simulink model "leftLaneChangeRestructuredTest"  (R2019b)
settings: Solver=FixedStepAuto  StartTime=0.0  StopTime=10.0  FixedStep=Ts_bp  RelTol=1e-3
values from neighbouring files (symbols this model uses):
  P_init = .001    (= 0.001)    [initialization.m]
  rel_x = 0    [initialization.m]
  Ts_bp = 0.1    [initialization.m]    (also in laneChangeSinusoidalFcn.m = 0.01; laneChangeSinusoidalJacobianFcn.m = 0.01; leftLaneChangeParametricFcn.m; leftLaneChangeParametricWithAccFcn.m = 0.01)
  vx = X(2)    [cv_model_fun.m]    (also in initialization.m = 10)
  vy = X(4)    [cv_model_fun.m]    (also in initialization.m = 0)
  x = X(1)    [KinematicBicycleModel.m]    (also in SimplifiedKinematicBicycleModel.m; behavior_model.m = 0:0.01:20; cca_model_fun.m; ctra_model_fun.m)
  y = X(2)    [KinematicBicycleModel.m]    (also in SimplifiedKinematicBicycleModel.m; behavior_model.m = [distances velocities]; cca_model_fun.m; ctra_model_fun.m)
undefined symbols (not defined in the file or in its folder): sigbuilder_block
libraries: simulink x2
settings Model: Creator=jasprit  LastModifiedBy=jasprit

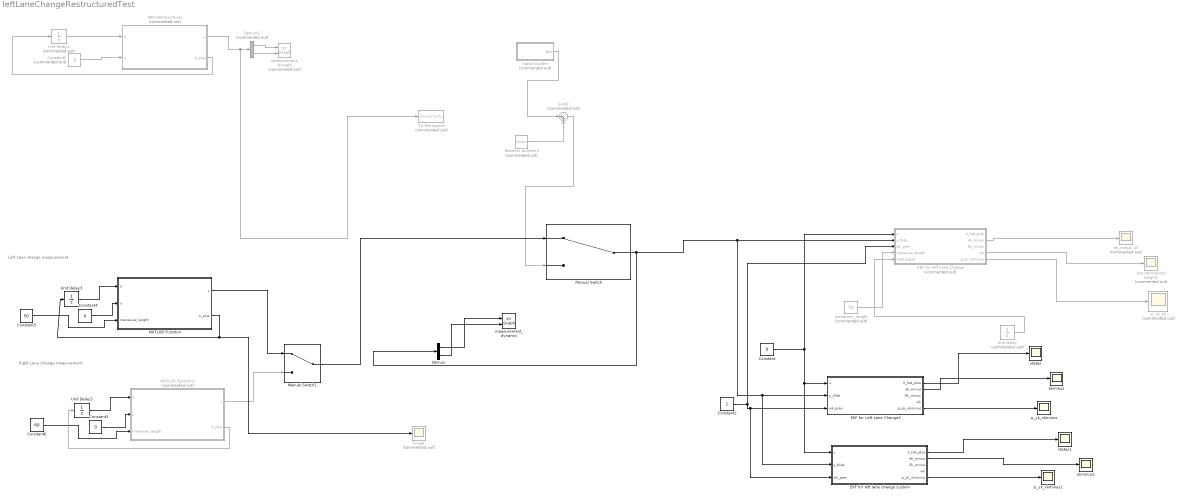
== system leftLaneChangeRestructuredTest ==
  note: Left Lane change measurement
  note: Right Lane Change measurement
  Constant : Constant  Value=0
  Constant1 : Constant  Value=0  SampleTime=-1
  Constant2 : Constant
  Constant3 : Constant  Value=50  SampleTime=-1
  Constant4 : Constant  Value=0  SampleTime=-1
  Constant5 : Constant  Commented=on  Value=0  SampleTime=-1
  Constant6 : Constant  Value=60
  Demux : Demux  Outputs=2
  Demux2 : Demux  Commented=on  Outputs=2
  EKF for Left Lane Change2 : Subsystem
  EKF for left Lane Change : Subsystem  Commented=on  TreatAsAtomicUnit=on
  EKF for left lane change custom : Subsystem
  MATLAB Function : MATLAB Function  TreatAsAtomicUnit=on
  MATLAB Function1 : MATLAB Function  Commented=on  TreatAsAtomicUnit=on
  MATLAB Function2 : MATLAB Function  Commented=on  TreatAsAtomicUnit=on
  Manual Switch : ManualSwitch
  Manual Switch1 : ManualSwitch
  Random Number2 : RandomNumber  Commented=on  Variance=0.0025  SampleTime=0.01
  Scope : Scope  Commented=on
  Signal Builder : Subsystem  Tag=STV Subsys  Commented=on  LoadFcn=sigbuilder_block('load');  StartFcn=sigbuilder_block('start');  StopFcn=sigbuilder_block('stop');  ClipboardFcn=sigbuilder_block('clipboard');  mask(Sigbuilder block){tuvar=[0:10]}
      mask help: Simulink:masks:SigbuilderBlock_MD
      mask init:
      | if ~strcmp(get_param(bdroot(gcbh),'SimulationStatus'),'stopped') tuvar = sigbuilder_block('maskInit'); end
      settings: CopyFcn=sigbuilder_block('copy');  DeleteFcn=sigbuilder_block('delete');  ModelCloseFcn=sigbuilder_block('modelClose');  PreSaveFcn=sigbuilder_block('preSave');  PauseFcn=sigbuilder_block('pause');  ContinueFcn=sigbuilder_block('continue');  NameChangeFcn=sigbuilder_block('namechange');  OpenFcn=sigbuilder_block('open',[418.5 99 558 422.25 ]);  CloseFcn=sigbuilder_block('close');
      mask Display: plot(0, 0, 100, 100,[2, 2, 32, 32, 2], [68, 8, 8, 68, 68],[32, 2], [38, 38], [32, 19, 2],[53, 60, 44], [32, 17, 17, 2],[16, 16, 31, 31]);txt = getActiveGroup(gcbh);text(2, 100, txt,'verticalAlignment', 'top');
  Sum2 : Sum  Commented=on  Inputs=|++
  To Workspace : ToWorkspace  Commented=on  VariableName=ground_truth_2  SaveFormat=Timeseries  SampleTime=-1
  Unit Delay : UnitDelay  Commented=on  SampleTime=-1  HasFrameUpgradeWarning=on
  Unit Delay3 : UnitDelay  InitialCondition=[x vx y vy]  SampleTime=Ts_bp  HasFrameUpgradeWarning=on
  Unit Delay4 : UnitDelay  Commented=on  InitialCondition=[x vx y vy]  SampleTime=-1  HasFrameUpgradeWarning=on
  Unit Delay5 : UnitDelay  InitialCondition=[x vx y vy]  SampleTime=Ts_bp  HasFrameUpgradeWarning=on
  ek_minus_All : Scope  Commented=on
  ekminus : Scope
  ekminus1 : Scope
  maneuver_length : Constant  Commented=on  Value=50
  measurement_dynamic : simulink/Sinks/XY Graph  xmin=-1  xmax=100  ymin=-5  ymax=5  st=-1
  measurement_straight : simulink/Sinks/XY Graph  Commented=on  xmin=-1  xmax=200  ymin=-5  ymax=5  st=-1
  p_yk_xk : Scope  Commented=on
  p_yk_xkminus : Scope
  p_yk_xkminus1 : Scope
  pre-normalized weights : Scope  Commented=on
  states : Scope
  states1 : Scope
  wires:
  Unit Delay3/1 -> MATLAB Function/1(X)
  MATLAB Function2/1(y) -> Manual Switch1/2
  Demux2/1 -> measurement_straight/1
  Constant/1 -> EKF for left lane change custom/1(u), EKF for Left Lane Change2/1(u), EKF for left Lane Change/1(u)
  Unit Delay5/1 -> MATLAB Function2/1(X)
  MATLAB Function1/1(y) -> To Workspace/1, Demux2/1
  Constant1/1 -> MATLAB Function2/2(u)
  Unit Delay/1 -> EKF for left Lane Change/5(reset signal)
  Constant2/1 -> EKF for left Lane Change/3(wk_prev), EKF for left lane change custom/3(wk_prev), EKF for Left Lane Change2/3(wk_prev)
  Constant6/1 -> MATLAB Function2/3(maneuver_length)
  MATLAB Function/1(y) -> Manual Switch1/1
  Manual Switch/1 -> EKF for left lane change custom/2(y_tilde), EKF for Left Lane Change2/2(y_tilde), EKF for left Lane Change/2(y_tilde), Demux/1
  Constant4/1 -> MATLAB Function/2(u)
  Unit Delay4/1 -> MATLAB Function1/1(X)
  Demux/1 -> measurement_dynamic/1
  Constant3/1 -> MATLAB Function/3(maneuver_length)
  MATLAB Function1/2(X_plus) -> Unit Delay4/1
  MATLAB Function/2(X_plus) -> Scope/1, Unit Delay3/1
  EKF for left Lane Change/5(p_yk_xkminus) -> p_yk_xk/1
  Sum2/1 -> Manual Switch/2
  Signal Builder/1(Bus) -> Sum2/1
  Random Number2/1 -> Sum2/2
  maneuver_length/1 -> EKF for left Lane Change/4(maneuver_length)
  EKF for left Lane Change/2(ek_minus) -> ek_minus_All/1
  Constant5/1 -> MATLAB Function1/2(u)
  MATLAB Function2/2(X_plus) -> Unit Delay5/1
  Demux2/2 -> measurement_straight/2
  Demux/2 -> measurement_dynamic/2
  EKF for left Lane Change/4(wk) -> pre-normalized weights/1
  Manual Switch1/1 -> Manual Switch/1
  EKF for Left Lane Change2/1(X_hat_plus) -> states/1
  EKF for Left Lane Change2/2(ek_minus) -> ekminus/1
  EKF for Left Lane Change2/5(p_yk_xkminus) -> p_yk_xkminus/1
  EKF for left lane change custom/2(ek_minus) -> ekminus1/1
  EKF for left lane change custom/1(X_hat_plus) -> states1/1
  EKF for left lane change custom/5(p_yk_xkminus) -> p_yk_xkminus1/1

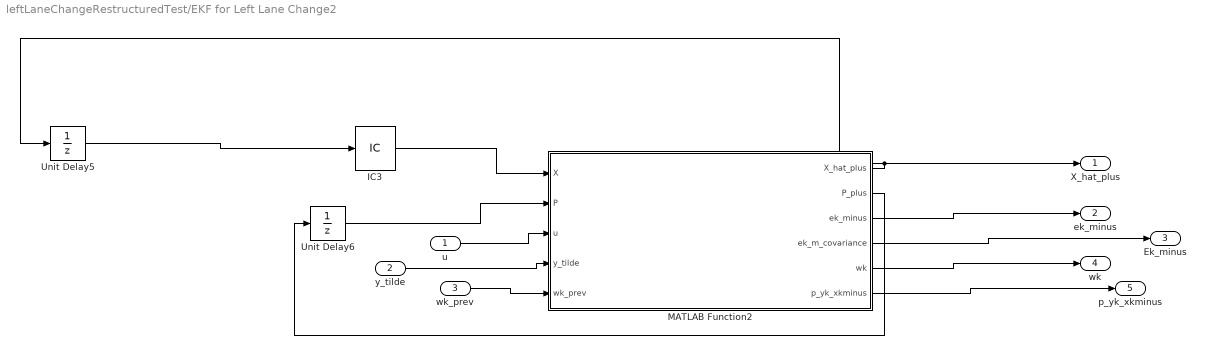
== system leftLaneChangeRestructuredTest/EKF for Left Lane Change2 ==
  u : Inport
  y_tilde : Inport  Port=2
  wk_prev : Inport  Port=3
  IC3 : InitialCondition  Value=[x vx y vy]
  MATLAB Function2 : MATLAB Function  TreatAsAtomicUnit=on
  Unit Delay5 : UnitDelay  SampleTime=-1  HasFrameUpgradeWarning=on
  Unit Delay6 : UnitDelay  InitialCondition=P_init  SampleTime=-1  HasFrameUpgradeWarning=on
  X_hat_plus : Outport  VectorParamsAs1DForOutWhenUnconnected=off
  ek_minus : Outport  Port=2  VectorParamsAs1DForOutWhenUnconnected=off
  Ek_minus : Outport  Port=3  VectorParamsAs1DForOutWhenUnconnected=off
  wk : Outport  Port=4  VectorParamsAs1DForOutWhenUnconnected=off
  p_yk_xkminus : Outport  Port=5  VectorParamsAs1DForOutWhenUnconnected=off
  wires:
  MATLAB Function2/2(P_plus) -> Unit Delay6/1
  u/1 -> MATLAB Function2/3(u)
  Unit Delay5/1 -> IC3/1
  y_tilde/1 -> MATLAB Function2/4(y_tilde)
  MATLAB Function2/1(X_hat_plus) -> Unit Delay5/1, X_hat_plus/1
  IC3/1 -> MATLAB Function2/1(X)
  Unit Delay6/1 -> MATLAB Function2/2(P)
  MATLAB Function2/3(ek_minus) -> ek_minus/1
  MATLAB Function2/4(ek_m_covariance) -> Ek_minus/1
  MATLAB Function2/5(wk) -> wk/1
  MATLAB Function2/6(p_yk_xkminus) -> p_yk_xkminus/1
  wk_prev/1 -> MATLAB Function2/5(wk_prev)

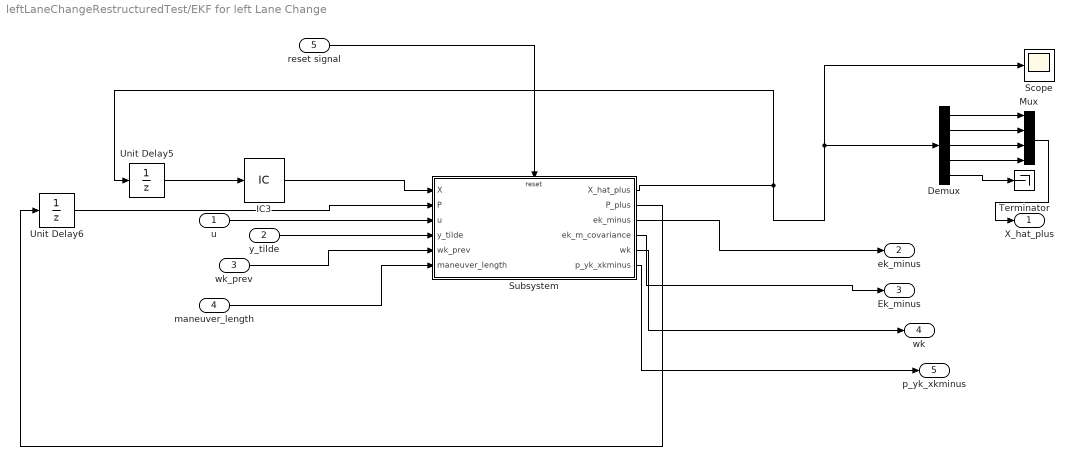
== system leftLaneChangeRestructuredTest/EKF for left Lane Change ==
  u : Inport
  y_tilde : Inport  Port=2
  wk_prev : Inport  Port=3
  maneuver_length : Inport  Port=4
  reset signal : Inport  Port=5
  Demux : Demux  Outputs=5
  IC3 : InitialCondition  Value=[x vx y vy rel_x]
  Mux : Mux
  Scope : Scope
  Subsystem : Subsystem
  Terminator : Terminator
  Unit Delay5 : UnitDelay  InitialCondition=[x vx y vy rel_x]  SampleTime=-1  HasFrameUpgradeWarning=on
  Unit Delay6 : UnitDelay  InitialCondition=diag([P_init, P_init, P_init, P_init, P_init])  SampleTime=-1  HasFrameUpgradeWarning=on
  X_hat_plus : Outport  VectorParamsAs1DForOutWhenUnconnected=off
  ek_minus : Outport  Port=2  VectorParamsAs1DForOutWhenUnconnected=off
  Ek_minus : Outport  Port=3  VectorParamsAs1DForOutWhenUnconnected=off
  wk : Outport  Port=4  VectorParamsAs1DForOutWhenUnconnected=off
  p_yk_xkminus : Outport  Port=5  VectorParamsAs1DForOutWhenUnconnected=off
  wires:
  Mux/1 -> X_hat_plus/1
  Demux/4 -> Mux/4
  Demux/5 -> Terminator/1
  Demux/3 -> Mux/3
  Demux/2 -> Mux/2
  Unit Delay5/1 -> IC3/1
  Demux/1 -> Mux/1
  Subsystem/1(X_hat_plus) -> Demux/1, Scope/1, Unit Delay5/1
  IC3/1 -> Subsystem/1(X)
  u/1 -> Subsystem/3(u)
  y_tilde/1 -> Subsystem/4(y_tilde)
  wk_prev/1 -> Subsystem/5(wk_prev)
  maneuver_length/1 -> Subsystem/6(maneuver_length)
  Subsystem/3(ek_minus) -> ek_minus/1
  Subsystem/4(ek_m_covariance) -> Ek_minus/1
  Subsystem/5(wk) -> wk/1
  Subsystem/6(p_yk_xkminus) -> p_yk_xkminus/1
  Unit Delay6/1 -> Subsystem/2(P)
  Subsystem/2(P_plus) -> Unit Delay6/1
  reset signal/1 -> Subsystem/Reset

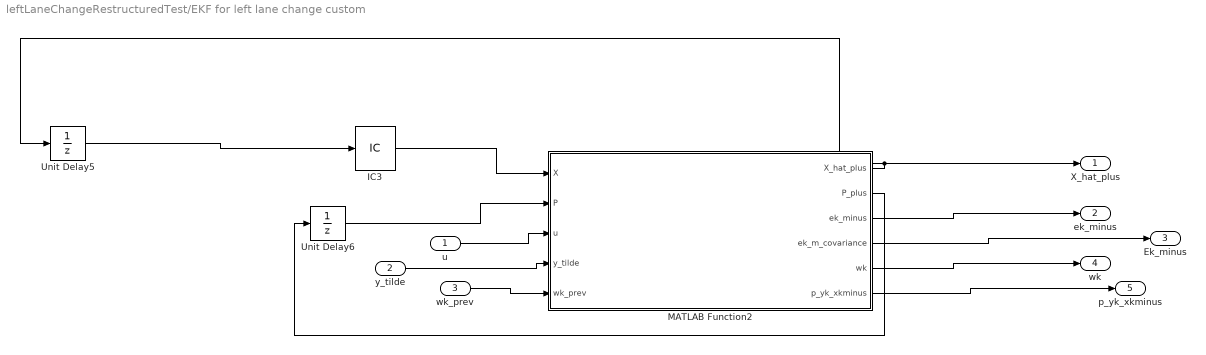
== system leftLaneChangeRestructuredTest/EKF for left lane change custom ==
  u : Inport
  y_tilde : Inport  Port=2
  wk_prev : Inport  Port=3
  IC3 : InitialCondition  Value=[x vx y vy]
  MATLAB Function2 : MATLAB Function  TreatAsAtomicUnit=on
  Unit Delay5 : UnitDelay  SampleTime=-1  HasFrameUpgradeWarning=on
  Unit Delay6 : UnitDelay  InitialCondition=P_init  SampleTime=-1  HasFrameUpgradeWarning=on
  X_hat_plus : Outport  VectorParamsAs1DForOutWhenUnconnected=off
  ek_minus : Outport  Port=2  VectorParamsAs1DForOutWhenUnconnected=off
  Ek_minus : Outport  Port=3  VectorParamsAs1DForOutWhenUnconnected=off
  wk : Outport  Port=4  VectorParamsAs1DForOutWhenUnconnected=off
  p_yk_xkminus : Outport  Port=5  VectorParamsAs1DForOutWhenUnconnected=off
  wires:
  MATLAB Function2/2(P_plus) -> Unit Delay6/1
  u/1 -> MATLAB Function2/3(u)
  Unit Delay5/1 -> IC3/1
  y_tilde/1 -> MATLAB Function2/4(y_tilde)
  MATLAB Function2/1(X_hat_plus) -> Unit Delay5/1, X_hat_plus/1
  IC3/1 -> MATLAB Function2/1(X)
  Unit Delay6/1 -> MATLAB Function2/2(P)
  MATLAB Function2/3(ek_minus) -> ek_minus/1
  MATLAB Function2/4(ek_m_covariance) -> Ek_minus/1
  MATLAB Function2/5(wk) -> wk/1
  MATLAB Function2/6(p_yk_xkminus) -> p_yk_xkminus/1
  wk_prev/1 -> MATLAB Function2/5(wk_prev)

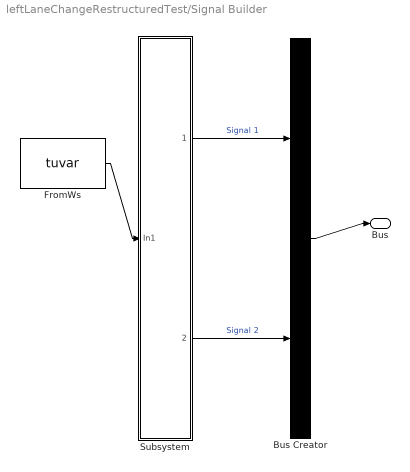
== system leftLaneChangeRestructuredTest/Signal Builder ==
  Bus Creator : BusCreator  Tag=Bus Creator  Inputs=2
  FromWs : FromWorkspace  Tag=STV FromWs  VariableName=tuvar  SampleTime=0
      SigBuilderData=|
      | common.afterFinalStr = 'Extrapolate'
      | common.sampleTime = 0
      | dataSet.timeRange = [0 20]
      | dataSet.name = 'Group 1'
      | sbobj.Groups.Name = 'Group 1'
      | sbobj.Groups.Signals(1).Name = 'Signal 1'
      | sbobj.Groups.Signals(1).XData = [0 0.01 0.02 0.03 0.04 0.05 0.06 0.07 0.08 0.09 0.1 0.11 ... (2001 elements, 1x2001)]
      | sbobj.Groups.Signals(1).YData = [0 0.1 0.2 0.3 0.4 0.5 0.6 0.7 0.8 0.9 1 1.1 ... (2001 elements, 1x2001)]
      | sbobj.Groups.Signals(2).Name = 'Signal 2'
      | sbobj.Groups.Signals(2).XData = [0 0.01 0.02 0.03 0.04 0.05 0.06 0.07 0.08 0.09 0.1 0.11 ... (2001 elements, 1x2001)]
      | sbobj.Groups.Signals(2).YData = [0 0 0 0 0 0 0 0 0 0 0 0 ... (2001 elements, 1x2001)]
      | sbobj.Groups.TimeRange = [0 20]
  Subsystem : Subsystem
  Bus : Outport  VectorParamsAs1DForOutWhenUnconnected=off
  wires:
  FromWs/1 -> Subsystem/1(In1)
  Bus Creator/1 -> Bus/1
  Subsystem/1(Signal 1) -> Bus Creator/1  "Signal 1"
  Subsystem/2(Signal 2) -> Bus Creator/2  "Signal 2"

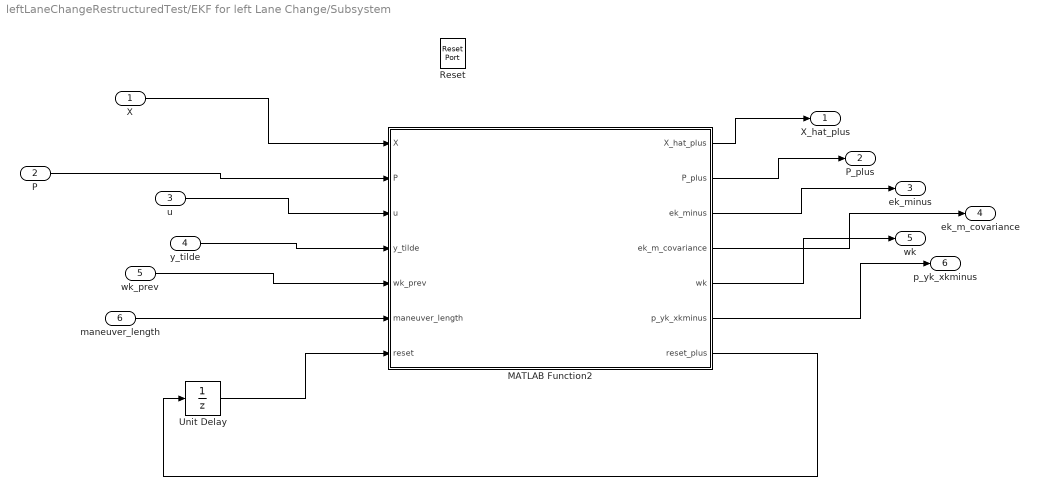
== system leftLaneChangeRestructuredTest/EKF for left Lane Change/Subsystem ==
  X : Inport
  P : Inport  Port=2
  u : Inport  Port=3
  y_tilde : Inport  Port=4
  wk_prev : Inport  Port=5
  maneuver_length : Inport  Port=6
  Reset : ResetPort  DisableCoverage=on
  MATLAB Function2 : MATLAB Function  TreatAsAtomicUnit=on
  Unit Delay : UnitDelay  InitialCondition=1  SampleTime=-1  HasFrameUpgradeWarning=on
  X_hat_plus : Outport  VectorParamsAs1DForOutWhenUnconnected=off
  P_plus : Outport  Port=2  VectorParamsAs1DForOutWhenUnconnected=off
  ek_minus : Outport  Port=3  VectorParamsAs1DForOutWhenUnconnected=off
  ek_m_covariance : Outport  Port=4  VectorParamsAs1DForOutWhenUnconnected=off
  wk : Outport  Port=5  VectorParamsAs1DForOutWhenUnconnected=off
  p_yk_xkminus : Outport  Port=6  VectorParamsAs1DForOutWhenUnconnected=off
  wires:
  MATLAB Function2/5(wk) -> wk/1
  MATLAB Function2/1(X_hat_plus) -> X_hat_plus/1
  X/1 -> MATLAB Function2/1(X)
  P/1 -> MATLAB Function2/2(P)
  u/1 -> MATLAB Function2/3(u)
  wk_prev/1 -> MATLAB Function2/5(wk_prev)
  MATLAB Function2/3(ek_minus) -> ek_minus/1
  y_tilde/1 -> MATLAB Function2/4(y_tilde)
  maneuver_length/1 -> MATLAB Function2/6(maneuver_length)
  MATLAB Function2/2(P_plus) -> P_plus/1
  MATLAB Function2/6(p_yk_xkminus) -> p_yk_xkminus/1
  MATLAB Function2/4(ek_m_covariance) -> ek_m_covariance/1
  Unit Delay/1 -> MATLAB Function2/7(reset)
  MATLAB Function2/7(reset_plus) -> Unit Delay/1

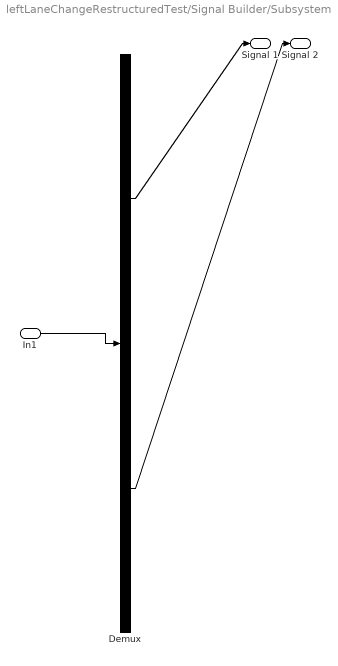
== system leftLaneChangeRestructuredTest/Signal Builder/Subsystem ==
  In1 : Inport
  Demux : Demux  Tag=STV Demux  Outputs=2
  Signal 1 : Outport  Tag=STV Outport  VectorParamsAs1DForOutWhenUnconnected=off
  Signal 2 : Outport  Tag=STV Outport  Port=2  VectorParamsAs1DForOutWhenUnconnected=off
  wires:
  In1/1 -> Demux/1
  Demux/1 -> Signal 1/1
  Demux/2 -> Signal 2/1

== matlab function leftLaneChangeRestructuredTest/EKF for Left Lane Change2/MATLAB Function2 ==
  data: X input; P input; u input; X_hat_plus output; y_tilde input; P_plus output; ek_minus output; ek_m_covariance output; wk output; p_yk_xkminus output; wk_prev input
function [X_hat_plus, P_plus, ek_minus, ek_m_covariance, wk, p_yk_xkminus] = EKFLeftLaneChangeCustom(X, P, u, y_tilde, wk_prev)

    maneuver_length = 50;  %meters
    lane_center_to_center_distance = 3.5;   %meters
    
    %%
    %TODO: See how can this be moved out of the function later
    %sampling time
    Ts = 0.1;

    % measurement noise covariance
%     R = [0.2 0; 0 0.2];
    R = [0.0025 0; 0 0.0025];
    
    % process noise covariance
%     Q = diag([0.5 5.0 0.5 5.0]);
    Q = diag([0.001 0.001 0.001 0.001]);

    % states - X = [x vx y vy] -     
    Ck = [1 0 0 0; 0 0 1 0];

    F = leftLaneChangeParametricJacobianFcn(X, u, maneuver_length, lane_center_to_center_distance);
    %%
    % Now estimate states using kalman filter
    
    %predict
    xhat_minus = leftLaneChangeParametricFcn(X, u, maneuver_length, lane_center_to_center_distance);
    P_minus = (F * P * F') + Ts*Q;
    yhat_minus = Ck * xhat_minus;

    %correct
    ek_minus = y_tilde - yhat_minus;    %residual
    ek_m_covariance = Ck * P_minus *Ck' + R;    %residual covariance
    K = P_minus * Ck' * inv(ek_m_covariance);
    X_hat_plus = xhat_minus + K * ek_minus;
    P_plus = (eye(4) - K * Ck) * P_minus;
    
    %calculate MMAE weights
    p_yk_xkminus = 1/sqrt(det(2*pi*ek_m_covariance))*exp(-1/2 * ek_minus'* inv(ek_m_covariance) * ek_minus);
    wk = wk_prev * p_yk_xkminus;

    
end

== matlab function leftLaneChangeRestructuredTest/EKF for left lane change custom/MATLAB Function2 ==
  data: X input; P input; u input; X_hat_plus output; y_tilde input; P_plus output; ek_minus output; ek_m_covariance output; wk output; p_yk_xkminus output; wk_prev input
function [X_hat_plus, P_plus, ek_minus, ek_m_covariance, wk, p_yk_xkminus] = EKFLeftLaneChangeCustom(X, P, u, y_tilde, wk_prev)

%%    
    persistent leftLCfilter;
    if isempty(leftLCfilter)
        maneuver_length = 50;  %meters
        lane_center_to_center_distance = 3.5;   %meters
        
        %TODO: See how can this be moved out of the function later
        %sampling time
        Ts = 0.1;
        
        mm = LeftLaneChangeSinusoidalMotionModel(Ts,maneuver_length, lane_center_to_center_distance);
        
        leftLCfilter = XKalmanFilter(Ts,mm);
        
        % measurement noise covariance
        %     R = [0.2 0; 0 0.2];
        R = [0.0025 0; 0 0.0025];
        
        % process noise covariance
        %     Q = diag([0.5 5.0 0.5 5.0]);
        Q = diag([0.001 0.001 0.001 0.001]);
        
        leftLCfilter.updateNoiseStatistics(Q, R);

    end
%%
    % Now estimate states using kalman filter
    %predict
    [Xhat_minus, P_minus] = leftLCfilter.predict(X, P, u);
    
    %correct
    [X_hat_plus, P_plus] = leftLCfilter.correct(y_tilde);
    ek_minus = leftLCfilter.err_innov;    %residual
    ek_m_covariance = leftLCfilter.err_cov;    %residual covariance
    
    %calculate MMAE weights
    p_yk_xkminus = leftLCfilter.likelihood;
    wk = wk_prev * p_yk_xkminus;
   
end

== matlab function leftLaneChangeRestructuredTest/EKF for left Lane Change/Subsystem/MATLAB Function2 ==
  data: X input; P input; u input; X_hat_plus output; y_tilde input; P_plus output; ek_minus output; ek_m_covariance output; wk output; p_yk_xkminus output; wk_prev input; maneuver_length input; reset input; reset_plus output
function [X_hat_plus, P_plus, ek_minus, ek_m_covariance, wk, p_yk_xkminus, reset_plus] = EKFLeftLaneChangeCustom(X, P, u, y_tilde, wk_prev, maneuver_length, reset)

    %%
    %TODO: See how can this be moved out of the function later
    %sampling time
    Ts_bp = 0.1;
%     maneuver_length = 150;  %m
    lane_center_to_center_distance = 3.5;   %meters

    % measurement noise covariance
%      R = [0.25 0; 0 0.25];
   R = [0.0025 0; 0 0.0025];
    
    % process noise covariance
%     Q = diag([0.5 5.0 0.5 5.0]);
    Q = diag([0.001 0.001 0.001 0.001 0.001]);

    % states - X = [x vx y vy] -     
    Ck = [1 0 0 0 0 ; 0 0 1 0 0];

    if reset == 1
        reset = 0;
        
        % x0 = x, update the initiation point to x and reset the covariance
        X(5) = X(1);
        P(5,5) = 50;
    end
    
    reset_plus = reset;
    
    F = leftLaneChangeRelativeJacobianFcn(X, u, maneuver_length, lane_center_to_center_distance);
    %%
    % Now estimate states using kalman filter
    
    %predict
    xhat_minus = leftLaneChangeRelativeFcn(X, u, maneuver_length, lane_center_to_center_distance);
    P_minus = (F * P * F') + Ts_bp*Q;
    yhat_minus = Ck * xhat_minus;

    %correct
    ek_minus = y_tilde - yhat_minus;    %residual
    ek_m_covariance = Ck * P_minus *Ck' + R;    %residual covariance
    K = P_minus * Ck' * inv(ek_m_covariance);
    X_hat_plus = xhat_minus + K * ek_minus;
    P_plus = (eye(5) - K * Ck) * P_minus;
    
    %calculate MMAE weights
    p_yk_xkminus = 1/sqrt(det(2*pi*ek_m_covariance))*exp(-1/2 * ek_minus'* inv(ek_m_covariance) * ek_minus);
    wk = wk_prev * p_yk_xkminus;

    
end

== matlab function leftLaneChangeRestructuredTest/MATLAB Function ==
  data: X input; u input; y output; X_plus output; maneuver_length input
function [y, X_plus]= measurementsForLaneChange(X, u, maneuver_length)

    Ts_bp = 0.1;
%     maneuver_length = 150;  %m
    lane_center_to_center_distance = 3.5;   %meters

    % states - X = [x vx y vy] -     
    Ck = [1 0 0 0; 0 0 1 0];

    % measurement noise std_dev
%     R_sigma = [0.5 0; 0 0.5];
   R_sigma = [0.05 0; 0 0.05];
    
    % process noise std dev
%    sigma_matrix = diag([0.16 0.16 0.16 0.16]);
    sigma_matrix = diag([0.032 0.032 0.032 0.032]);
    
%     if t < 15
%         Ak = [1 Ts 0 0; 0 1 0 0; 0 0 1 Ts; 0 0 0 1];
%         Bk = 0;
%         X_plus = Ak * X + Bk * u + sqrt(Ts) * sigma_matrix * randn(4,1);
%     else
        X_plus = leftLaneChangeParametricFcn(X, u, maneuver_length, lane_center_to_center_distance) + sqrt(Ts_bp)*sigma_matrix*randn(4,1);    
%     end
    
    y = Ck * X_plus + R_sigma * randn(2,1);
    
end

== matlab function leftLaneChangeRestructuredTest/MATLAB Function1 ==
  data: X input; u input; y output; X_plus output
function [y, X_plus]= measurementsForStraightMotion(X, u)

    Ts_bp = 0.01;
    % states - X = [x vx y vy] -     
    Ak = [1 Ts_bp 0 0; 0 1 0 0; 0 0 1 Ts_bp; 0 0 0 1];
    Bk = 0;
    Ck = [1 0 0 0; 0 0 1 0];

    % measurement noise std_dev
%     R_sigma = [0.5 0; 0 0.5];
   R_sigma = [0.05 0; 0 0.05];
    
    % process noise std dev
%    sigma_matrix = diag([0.16 0.16 0.16 0.16]);
    sigma_matrix = diag([0.032 0.032 0.032 0.032]);
  
    X(3) = 0;
%    X(4) = 0;
    
    X_plus = Ak * X + Bk * u + sqrt(Ts_bp)*sigma_matrix*randn(4,1);    
    
    y = Ck * X_plus + R_sigma * randn(2,1);
    
end

== matlab function leftLaneChangeRestructuredTest/MATLAB Function2 ==
  data: X input; u input; y output; X_plus output; maneuver_length input
function [y, X_plus]= measurementsForLaneChange(X, u, maneuver_length)

    Ts_bp = 0.01;
%    maneuver_length = 150;  %m
    lane_center_to_center_distance = 3.5;   %meters

    % states - X = [x vx y vy] -     
    Ck = [1 0 0 0; 0 0 1 0];

    % measurement noise std_dev
%     R_sigma = [0.5 0; 0 0.5];
   R_sigma = [0.05 0; 0 0.05];
    
    % process noise std dev
%    sigma_matrix = diag([0.16 0.16 0.16 0.16]);
    sigma_matrix = diag([0.032 0.032 0.032 0.032]);
    
%     if t < 15
%         Ak = [1 Ts 0 0; 0 1 0 0; 0 0 1 Ts; 0 0 0 1];
%         Bk = 0;
%         X_plus = Ak * X + Bk * u + sqrt(Ts) * sigma_matrix * randn(4,1);
%     else
        X_plus = rightLaneChangeParametricFcn(X, u, maneuver_length, lane_center_to_center_distance) + sqrt(Ts_bp)*sigma_matrix*randn(4,1);    
%     end
    
    y = Ck * X_plus + R_sigma * randn(2,1);
    
end
